simulink model "PV_battery_converter_simulation"  (Simulink 7.8)
settings: Solver=ode45  StartTime=0.0  StopTime=3600*14  FixedStep=0.01  RelTol=1e-3
values from neighbouring files (symbols this model uses):
  G_vec = [min(G_log(:,2)):(max(G_log(:,2)) - min(G_log(:,2)))/49:max(G_log(:,2))]/1000    [make_pv_characteristics_table.m]
  Ppv_to_Ipv = [Ppv_to_Ipv(:,:,2) Ppv_to_Ipv(:,:,3)]    [make_pv_characteristics_table.m]
undefined symbols (not defined in the file or in its folder): Ppv_vec
libraries: simulink x2
settings Model: Creator=dhshin  LastModifiedBy=dhshin

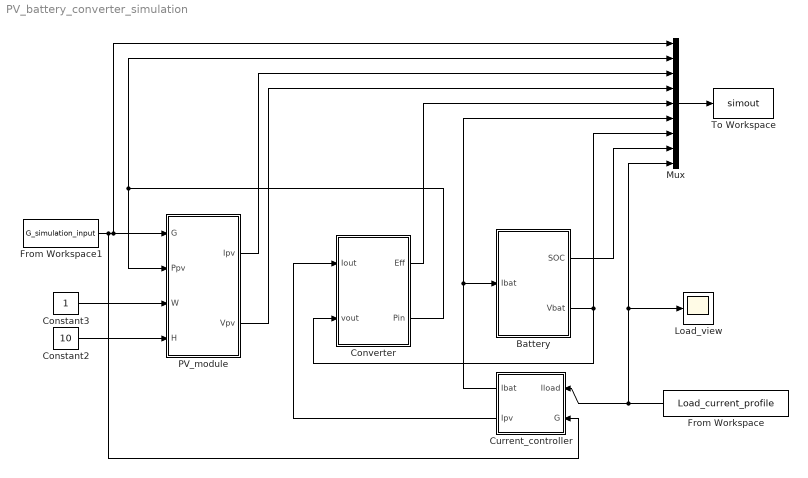
== system PV_battery_converter_simulation ==
  Battery : Subsystem
  Constant2 : Constant  Value=10
  Constant3 : Constant
  Converter : Subsystem
  Current_controller : Subsystem
  From Workspace : FromWorkspace  VariableName=Load_current_profile  SampleTime=0
  From Workspace1 : FromWorkspace  VariableName=G_simulation_input  SampleTime=0
  Load_view : Scope
      settings: TimeRange=100000  YMin=12.5  YMax=17  SaveName=ScopeData6
  Mux : Mux  Inputs=9
  PV_module : Subsystem
  To Workspace : ToWorkspace  VariableName=simout  SampleTime=-1  SaveFormat=Structure
  wires:
  From Workspace1/1 -> PV_module/1(G), Mux/1, Current_controller/2(G)
  Mux/1 -> To Workspace/1
  Constant2/1 -> PV_module/4(H)
  Constant3/1 -> PV_module/3(W)
  From Workspace/1 -> Current_controller/1(Iload), Mux/9, Load_view/1
  Current_controller/1(Ibat) -> Battery/1(Ibat), Mux/6
  Current_controller/2(Ipv) -> Converter/1(Iout)
  Battery/2(Vbat) -> Mux/7, Converter/2(vout)
  PV_module/2(Vpv) -> Mux/4
  Converter/2(Pin) -> PV_module/2(Ppv), Mux/2
  PV_module/1(Ipv) -> Mux/3
  Converter/1(Eff) -> Mux/5
  Battery/1(SOC) -> Mux/8

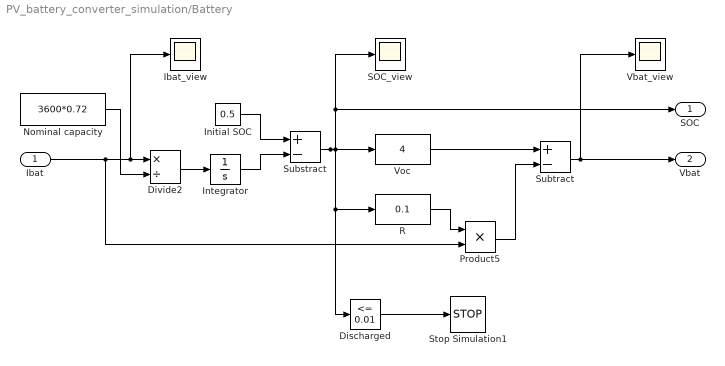
== system PV_battery_converter_simulation/Battery ==
  Ibat : Inport
  Discharged : simulink/Logic and Bit Operations/Compare To Constant  relop=<=  const=0.01  OutDataTypeStr=boolean  ZeroCross=off
  Divide2 : Product  Inputs=*/
  Ibat_view : Scope
      settings: TimeRange=100000  YMin=12.5  YMax=17  SaveName=ScopeData8
  Initial SOC : Constant  Value=0.5
  Integrator : Integrator
  Nominal capacity : Constant  Value=3600*0.72
  Product5 : Product  RndMeth=Zero
  R : Fcn  Expr=0.1
  SOC_view : Scope
      settings: SaveName=ScopeData2
  Stop Simulation1 : Stop
  Substract : Sum  Inputs=+-
  Subtract : Sum  Inputs=+-
  Vbat_view : Scope
      settings: TimeRange=100000  YMin=12.5  YMax=17
  Voc : Fcn  Expr=4
  SOC : Outport
  Vbat : Outport  Port=2
  wires:
  Ibat/1 -> Product5/2, Divide2/1, Ibat_view/1
  Substract/1 -> Voc/1, SOC_view/1, SOC/1, R/1, Discharged/1
  Product5/1 -> Subtract/2
  Subtract/1 -> Vbat/1, Vbat_view/1
  R/1 -> Product5/1
  Voc/1 -> Subtract/1
  Nominal capacity/1 -> Divide2/2
  Divide2/1 -> Integrator/1
  Integrator/1 -> Substract/2
  Initial SOC/1 -> Substract/1
  Discharged/1 -> Stop Simulation1/1

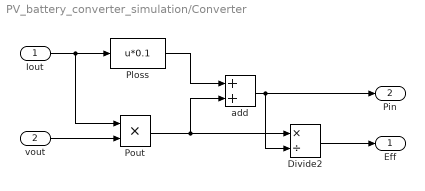
== system PV_battery_converter_simulation/Converter ==
  Iout : Inport
  vout : Inport  Port=2
  Divide2 : Product  Inputs=*/
  Ploss : Fcn  Expr=u*0.1
  Pout : Product  RndMeth=Zero
  add : Sum
  Eff : Outport
  Pin : Outport  Port=2
  wires:
  Iout/1 -> Ploss/1, Pout/1
  vout/1 -> Pout/2
  Ploss/1 -> add/1
  Pout/1 -> add/2, Divide2/1
  add/1 -> Divide2/2, Pin/1
  Divide2/1 -> Eff/1

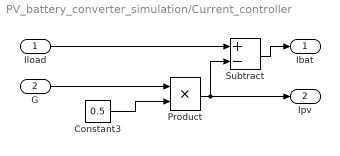
== system PV_battery_converter_simulation/Current_controller ==
  Iload : Inport
  G : Inport  Port=2
  Constant3 : Constant  Value=0.5
  Product : Product  RndMeth=Zero
  Subtract : Sum  Inputs=+-
  Ibat : Outport
  Ipv : Outport  Port=2
  wires:
  Product/1 -> Ipv/1, Subtract/2
  G/1 -> Product/1
  Constant3/1 -> Product/2
  Iload/1 -> Subtract/1
  Subtract/1 -> Ibat/1

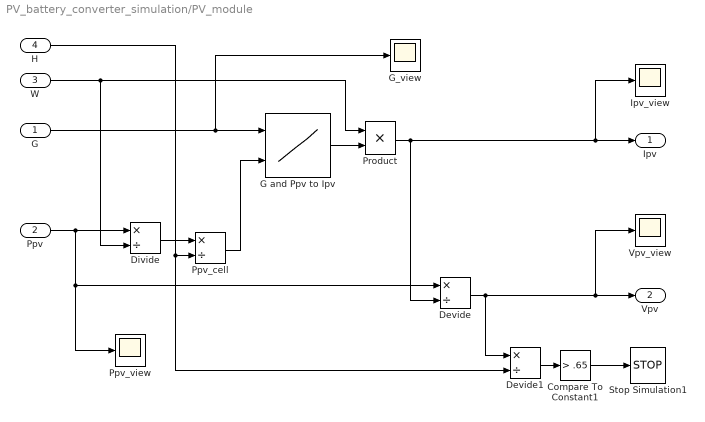
== system PV_battery_converter_simulation/PV_module ==
  G : Inport
  Ppv : Inport  Port=2
  W : Inport  Port=3
  H : Inport  Port=4
  Compare To Constant1 : simulink/Logic and Bit Operations/Compare To Constant  relop=>  const=.65  OutDataTypeStr=boolean  ZeroCross=off
  Devide : Product  Inputs=*/
  Devide1 : Product  Inputs=*/
  Divide : Product  Inputs=*/
  G and Ppv to Ipv : Lookup_n-D  BreakpointsForDimension1=G_vec  BreakpointsForDimension2=Ppv_vec  Table=Ppv_to_Ipv  RndMeth=Simplest  InputSameDT=on
  G_view : Scope
      settings: TimeRange=52200  YMin=0.955  YMax=1.02
  Ipv_view : Scope
      settings: TimeRange=100000  YMin=-2  YMax=12  SaveName=ScopeData3
  Ppv_cell : Product  Inputs=*/
  Ppv_view : Scope
      settings: TimeRange=100000  YMin=-2  YMax=12  SaveName=ScopeData5
  Product : Product  RndMeth=Zero
  Stop Simulation1 : Stop
  Vpv_view : Scope
      settings: TimeRange=100000  YMin=7  YMax=12  SaveName=ScopeData4
  Ipv : Outport
  Vpv : Outport  Port=2
  wires:
  Compare To Constant1/1 -> Stop Simulation1/1
  G/1 -> G and Ppv to Ipv/1, G_view/1
  G and Ppv to Ipv/1 -> Product/2
  Product/1 -> Devide/2, Ipv/1, Ipv_view/1
  Ppv/1 -> Divide/1, Devide/1, Ppv_view/1
  Ppv_cell/1 -> G and Ppv to Ipv/2
  Divide/1 -> Ppv_cell/1
  W/1 -> Divide/2, Product/1
  H/1 -> Ppv_cell/2, Devide1/2
  Devide/1 -> Vpv/1, Vpv_view/1, Devide1/1
  Devide1/1 -> Compare To Constant1/1
